simulink model "DAC_SIM_HL"  (R2017b)
settings: Solver=VariableStepDiscrete  StartTime=0.0  StopTime=N/Fs  RelTol=1e-3  EnableMultiTasking=on
values from neighbouring files (symbols this model uses):
  A = 0.5*(2-1)    (= 0.5)    [Model.m]
  ftest = 9e6    (= 9000000)    [Model.m]
  Tpass = 1/Fpass    (= 3.25520833333e-08)    [Model.m]
undefined symbols (not defined in the file or in its folder): a1, a2, a3, a4, b1, b2, b3, b4, g1, g2, g3, g4
libraries: dspmlti4 x3, dspsigops x2, simulink x1, dspsrcs4 x1
settings Model: Creator=o_cotte  LastModifiedBy=o_cotte
settings DataIOCC: LimitDataPoints=on  SaveFormat=Array
settings OptimizationCC: LifeSpan=inf
settings DebuggingCC: UnderspecifiedInitializationDetection=Classic  MergeDetectMultiDrivingBlocksExec=none  SolverPrmCheckMsg=warning  SFUnexpectedBacktrackingDiag=warning  SFNoUnconditionalDefaultTransitionDiag=warning  SFExecutionAtInitializationDiag=none
settings HardwareCC: ProdBitPerPointer=32  ProdBitPerSizeT=32  ProdBitPerPtrDiffT=32  ProdLargestAtomicFloat=None  ProdIntDivRoundTo=Undefined  ProdEndianess=Unspecified  ProdWordSize=32  ProdHWDeviceType=32-bit Generic
settings ModelReferenceCC: PropagateSignalLabelsOutOfModel=off
settings CodeAppCC: StateflowObjectComments=on
settings GRTTargetCC: TargetLangStandard=C89/C90 (ANSI)  GeneratePreprocessorConditionals=Disable all
settings ConfigComp: CovMetricSettings=dw  CovHtmlReporting=on  CovSaveCumulativeToWorkspaceVar=on  CovSaveSingleToWorkspaceVar=on  CovExternalEMLEnable=off

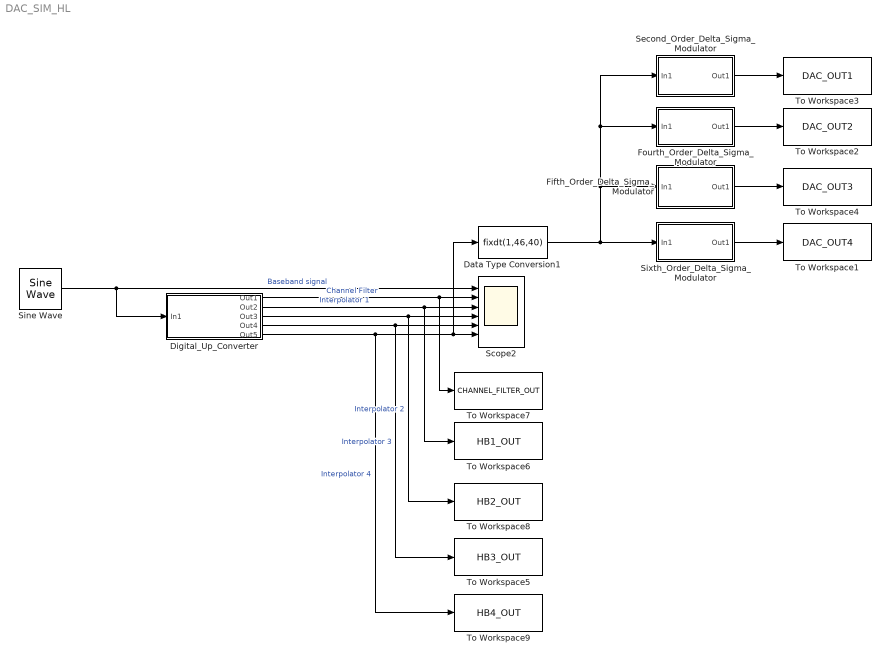
== system DAC_SIM_HL ==
  Data Type Conversion1 : DataTypeConversion  OutDataTypeStr=fixdt(1,46,40)  LockScale=on
  Digital_Up_Converter : Subsystem
  Fifth_Order_Delta_Sigma_Modulator : Subsystem
  Fourth_Order_Delta_Sigma_Modulator : Subsystem
  Scope2 : Scope  NumInputPorts=6
  Second_Order_Delta_Sigma_Modulator : Subsystem
  Sine Wave : dspsrcs4/Sine Wave  Amplitude=A  Frequency=ftest  Phase=0  SampleMode=Discrete  OutComplex=Real  CompMethod=Trigonometric fcn  TableSize=Speed  SampleTime=Tpass  SamplesPerFrame=1  ResetState=Restart at time zero  OutputFrames=on  dataType=double  wordLen=16  udDataType=sfix(16)  fracBitsMode=Best precision  numFracBits=15  OutDataTypeStr=double  LastOutDataTypeStr=double
  Sixth_Order_Delta_Sigma_Modulator : Subsystem
  To Workspace1 : ToWorkspace  VariableName=DAC_OUT4  SampleTime=-1
  To Workspace2 : ToWorkspace  VariableName=DAC_OUT2  SampleTime=-1
  To Workspace3 : ToWorkspace  VariableName=DAC_OUT1  SampleTime=-1
  To Workspace4 : ToWorkspace  VariableName=DAC_OUT3  SampleTime=-1
  To Workspace5 : ToWorkspace  VariableName=HB3_OUT  SampleTime=-1
  To Workspace6 : ToWorkspace  VariableName=HB1_OUT  SampleTime=-1
  To Workspace7 : ToWorkspace  VariableName=CHANNEL_FILTER_OUT  SampleTime=-1
  To Workspace8 : ToWorkspace  VariableName=HB2_OUT  SampleTime=-1
  To Workspace9 : ToWorkspace  VariableName=HB4_OUT  SampleTime=-1
  wires:
  Sine Wave/1 -> Digital_Up_Converter/1(In1), Scope2/1  "Baseband signal"
  Second_Order_Delta_Sigma_Modulator/1(Out1) -> To Workspace3/1
  Fourth_Order_Delta_Sigma_Modulator/1(Out1) -> To Workspace2/1
  Fifth_Order_Delta_Sigma_Modulator/1(Out1) -> To Workspace4/1
  Sixth_Order_Delta_Sigma_Modulator/1(Out1) -> To Workspace1/1
  Data Type Conversion1/1 -> Second_Order_Delta_Sigma_Modulator/1(In1), Fourth_Order_Delta_Sigma_Modulator/1(In1), Fifth_Order_Delta_Sigma_Modulator/1(In1), Sixth_Order_Delta_Sigma_Modulator/1(In1)
  Digital_Up_Converter/5(Out5) -> To Workspace9/1, Scope2/6, Data Type Conversion1/1  "Interpolator 4"
  Digital_Up_Converter/1(Out1) -> To Workspace7/1, Scope2/2  "Channel Filter"
  Digital_Up_Converter/2(Out2) -> To Workspace6/1, Scope2/3  "Interpolator 1"
  Digital_Up_Converter/3(Out3) -> To Workspace8/1, Scope2/4  "Interpolator 2"
  Digital_Up_Converter/4(Out4) -> To Workspace5/1, Scope2/5  "Interpolator 3"

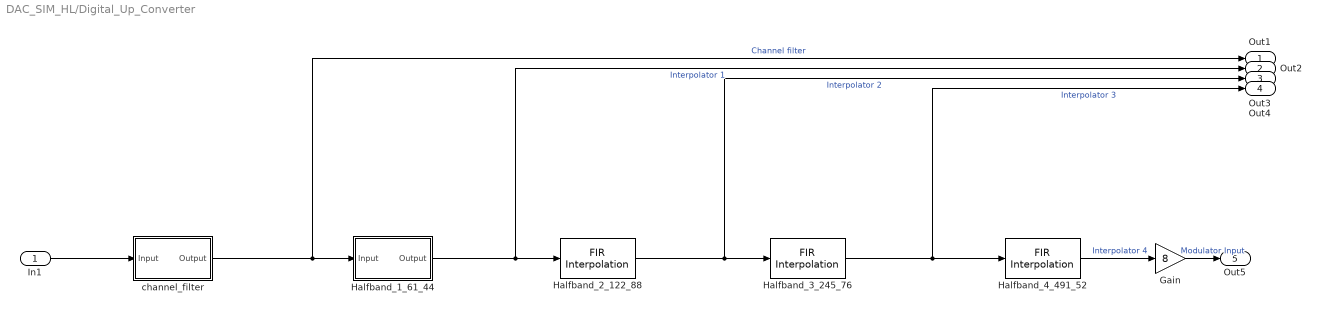
== system DAC_SIM_HL/Digital_Up_Converter ==
  In1 : Inport
  Gain : Gain  Gain=8
  Halfband_1_61_44 : Subsystem  Tag=FilterWizardSubSystem
      settings: ErrorFcn=dspFilterRealizedInBasicElemsAlgLoopErrFcnCallback
  Halfband_2_122_88 : dspmlti4/FIR Interpolation  Tag=BlockMethodSubSystem  FilterSource=Dialog parameters  h=[0.0076603622763803236 0 -0.053660411625164647 0 0.29602584582284724 0.5 0.29602584582284724 0 -0.053660411625164647 0 0.0076603622763803236]  L=2  FilterObject=Hm_firinterp  framing=Allow multirate processing  outputBufInitCond=0  roundingMode=Floor  overflowMode=off  firstCoeffDataTypeStr=Inherit: Same word length as input  firstCoeffMin=[]  firstCoeffMax=[]  firstCoeffLastDataTypeStr=Inherit: Same word length as input  outputDataTypeStr=Inherit: Same as accumulator  outputMin=[]  outputMax=[]  outputLastDataTypeStr=Inherit: Same as accumulator
      settings: SourceProductName=DSP System Toolbox
  Halfband_3_245_76 : dspmlti4/FIR Interpolation  Tag=BlockMethodSubSystem  FilterSource=Dialog parameters  h=[-0.032520171835777864 0 0.28248678153183715 0.5 0.28248678153183715 0 -0.032520171835777864]  L=2  FilterObject=Hm_firinterp  framing=Allow multirate processing  outputBufInitCond=0  roundingMode=Floor  overflowMode=off  firstCoeffDataTypeStr=Inherit: Same word length as input  firstCoeffMin=[]  firstCoeffMax=[]  firstCoeffLastDataTypeStr=Inherit: Same word length as input  outputDataTypeStr=Inherit: Same as accumulator  outputMin=[]  outputMax=[]  outputLastDataTypeStr=Inherit: Same as accumulator
      settings: SourceProductName=DSP System Toolbox
  Halfband_4_491_52 : dspmlti4/FIR Interpolation  Tag=BlockMethodSubSystem  FilterSource=Dialog parameters  h=[-0.031562027713033632 0 0.2815599679676668 0.5 0.2815599679676668 0 -0.031562027713033632]  L=2  FilterObject=Hm_firinterp  framing=Allow multirate processing  outputBufInitCond=0  roundingMode=Floor  overflowMode=off  firstCoeffDataTypeStr=Inherit: Same word length as input  firstCoeffMin=[]  firstCoeffMax=[]  firstCoeffLastDataTypeStr=Inherit: Same word length as input  outputDataTypeStr=Inherit: Same as accumulator  outputMin=[]  outputMax=[]  outputLastDataTypeStr=Inherit: Same as accumulator
      settings: SourceProductName=DSP System Toolbox
  channel_filter : Subsystem  Tag=FilterWizardSubSystem
      settings: ErrorFcn=dspFilterRealizedInBasicElemsAlgLoopErrFcnCallback
  Out1 : Outport
  Out2 : Outport  Port=2
  Out3 : Outport  Port=3
  Out4 : Outport  Port=4
  Out5 : Outport  Port=5
  wires:
  In1/1 -> channel_filter/1(Input)
  Halfband_1_61_44/1(Output) -> Out2/1, Halfband_2_122_88/1  "Interpolator 1"
  Halfband_2_122_88/1 -> Out3/1, Halfband_3_245_76/1  "Interpolator 2"
  Halfband_4_491_52/1 -> Gain/1  "Interpolator 4"
  Halfband_3_245_76/1 -> Out4/1, Halfband_4_491_52/1  "Interpolator 3"
  Gain/1 -> Out5/1  "Modulator Input"
  channel_filter/1(Output) -> Out1/1, Halfband_1_61_44/1(Input)  "Channel filter"

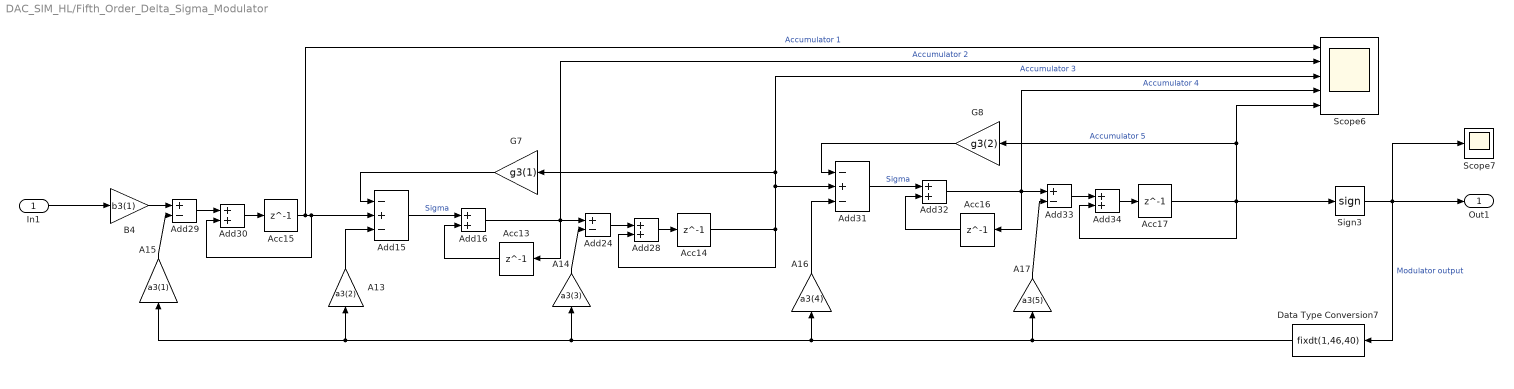
== system DAC_SIM_HL/Fifth_Order_Delta_Sigma_Modulator ==
  In1 : Inport
  A13 : Gain  Gain=a3(2)  OutDataTypeStr=Inherit: Same as input  ParamDataTypeStr=Inherit: Same as input  LockScale=on
  A14 : Gain  Gain=a3(3)  OutDataTypeStr=Inherit: Same as input  ParamDataTypeStr=Inherit: Same as input  LockScale=on
  A15 : Gain  Gain=a3(1)  OutDataTypeStr=Inherit: Same as input  ParamDataTypeStr=Inherit: Same as input  LockScale=on
  A16 : Gain  Gain=a3(4)  OutDataTypeStr=Inherit: Same as input  ParamDataTypeStr=Inherit: Same as input  LockScale=on
  A17 : Gain  Gain=a3(5)  OutDataTypeStr=Inherit: Same as input  ParamDataTypeStr=Inherit: Same as input  LockScale=on
  Acc{13..17} (5 alike) : Delay  DelayLength=1  InitialCondition=0
  Add15 : Sum  Inputs=-+-  SaturateOnIntegerOverflow=on  InputSameDT=on  OutDataTypeStr=Inherit: Same as first input
  Add{16,28,30,32,34} (5 alike) : Sum  Inputs=2  SaturateOnIntegerOverflow=on  InputSameDT=on  OutDataTypeStr=Inherit: Same as first input
  Add24 : Sum  Inputs=+-  SaturateOnIntegerOverflow=on  InputSameDT=on  OutDataTypeStr=Inherit: Same as first input
  Add29 : Sum  Inputs=+-  SaturateOnIntegerOverflow=on  InputSameDT=on  OutDataTypeStr=Inherit: Same as first input
  Add31 : Sum  Inputs=-+-  SaturateOnIntegerOverflow=on  InputSameDT=on  OutDataTypeStr=Inherit: Same as first input
  Add33 : Sum  Inputs=+-  SaturateOnIntegerOverflow=on  InputSameDT=on  OutDataTypeStr=Inherit: Same as first input
  B4 : Gain  Gain=b3(1)  OutDataTypeStr=Inherit: Same as input  ParamDataTypeStr=Inherit: Same as input  LockScale=on
  Data Type Conversion7 : DataTypeConversion  OutDataTypeStr=fixdt(1,46,40)  LockScale=on
  G7 : Gain  Gain=g3(1)  OutDataTypeStr=Inherit: Same as input  ParamDataTypeStr=Inherit: Same as input  LockScale=on
  G8 : Gain  Gain=g3(2)  OutDataTypeStr=Inherit: Same as input  ParamDataTypeStr=Inherit: Same as input  LockScale=on
  Scope6 : Scope  NumInputPorts=5
  Scope7 : Scope
  Sign3 : Signum
  Out1 : Outport
  wires:
  Acc16/1 -> Add32/2
  A16/1 -> Add31/3
  Add33/1 -> Add34/1
  G8/1 -> Add31/1
  Data Type Conversion7/1 -> A17/1, A14/1, A15/1, A13/1, A16/1
  A17/1 -> Add33/2
  Add31/1 -> Add32/1  "Sigma"
  Acc17/1 -> Sign3/1, Add34/2, Scope6/5, G8/1  "Accumulator 5"
  Add32/1 -> Scope6/4, Add33/1, Acc16/1  "Accumulator 4"
  Add34/1 -> Acc17/1
  Add24/1 -> Add28/1
  Acc13/1 -> Add16/2
  Add29/1 -> Add30/1
  Add30/1 -> Acc15/1
  A13/1 -> Add15/3
  Sign3/1 -> Scope7/1, Out1/1, Data Type Conversion7/1  "Modulator output"
  In1/1 -> B4/1
  Add16/1 -> Scope6/2, Add24/1, Acc13/1  "Accumulator 2"
  A15/1 -> Add29/2
  G7/1 -> Add15/1
  Acc14/1 -> Add31/2, Scope6/3, G7/1, Add28/2  "Accumulator 3"
  Add28/1 -> Acc14/1
  A14/1 -> Add24/2
  Acc15/1 -> Scope6/1, Add15/2, Add30/2  "Accumulator 1"
  Add15/1 -> Add16/1  "Sigma"
  B4/1 -> Add29/1

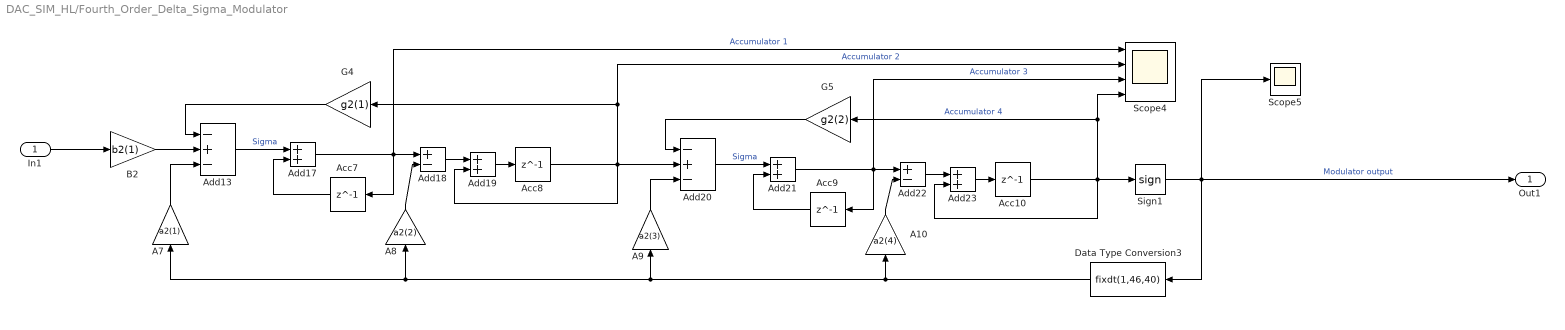
== system DAC_SIM_HL/Fourth_Order_Delta_Sigma_Modulator ==
  In1 : Inport
  A10 : Gain  Gain=a2(4)  OutDataTypeStr=Inherit: Same as input  ParamDataTypeStr=Inherit: Same as input  LockScale=on
  A7 : Gain  Gain=a2(1)  OutDataTypeStr=Inherit: Same as input  ParamDataTypeStr=Inherit: Same as input  LockScale=on
  A8 : Gain  Gain=a2(2)  OutDataTypeStr=Inherit: Same as input  ParamDataTypeStr=Inherit: Same as input  LockScale=on
  A9 : Gain  Gain=a2(3)  OutDataTypeStr=Inherit: Same as input  ParamDataTypeStr=Inherit: Same as input  LockScale=on
  Acc{7..10} (4 alike) : Delay  DelayLength=1  InitialCondition=0
  Add13 : Sum  Inputs=-+-  SaturateOnIntegerOverflow=on  InputSameDT=on  OutDataTypeStr=Inherit: Same as first input
  Add{17,19,21,23} (4 alike) : Sum  Inputs=2  SaturateOnIntegerOverflow=on  InputSameDT=on  OutDataTypeStr=Inherit: Same as first input
  Add18 : Sum  Inputs=+-  SaturateOnIntegerOverflow=on  InputSameDT=on  OutDataTypeStr=Inherit: Same as first input
  Add20 : Sum  Inputs=-+-  SaturateOnIntegerOverflow=on  InputSameDT=on  OutDataTypeStr=Inherit: Same as first input
  Add22 : Sum  Inputs=+-  SaturateOnIntegerOverflow=on  InputSameDT=on  OutDataTypeStr=Inherit: Same as first input
  B2 : Gain  Gain=b2(1)  OutDataTypeStr=Inherit: Same as input  ParamDataTypeStr=Inherit: Same as input  LockScale=on
  Data Type Conversion3 : DataTypeConversion  OutDataTypeStr=fixdt(1,46,40)  LockScale=on
  G4 : Gain  Gain=g2(1)  OutDataTypeStr=Inherit: Same as input  ParamDataTypeStr=Inherit: Same as input  LockScale=on
  G5 : Gain  Gain=g2(2)  OutDataTypeStr=Inherit: Same as input  ParamDataTypeStr=Inherit: Same as input  LockScale=on
  Scope4 : Scope  NumInputPorts=4
  Scope5 : Scope
  Sign1 : Signum
  Out1 : Outport
  wires:
  Sign1/1 -> Out1/1, Data Type Conversion3/1, Scope5/1  "Modulator output"
  Add13/1 -> Add17/1  "Sigma"
  In1/1 -> B2/1
  Data Type Conversion3/1 -> A10/1, A9/1, A7/1, A8/1
  B2/1 -> Add13/2
  Add17/1 -> Scope4/1, Add18/1, Acc7/1  "Accumulator 1"
  Acc8/1 -> Add20/2, Add19/2, Scope4/2, G4/1  "Accumulator 2"
  A7/1 -> Add13/3
  Acc7/1 -> Add17/2
  Acc10/1 -> Sign1/1, Scope4/4, G5/1, Add23/2  "Accumulator 4"
  Add19/1 -> Acc8/1
  Add18/1 -> Add19/1
  Add22/1 -> Add23/1
  G5/1 -> Add20/1
  Add23/1 -> Acc10/1
  Add21/1 -> Acc9/1, Scope4/3, Add22/1  "Accumulator 3"
  A10/1 -> Add22/2
  A8/1 -> Add18/2
  A9/1 -> Add20/3
  G4/1 -> Add13/1
  Add20/1 -> Add21/1  "Sigma"
  Acc9/1 -> Add21/2

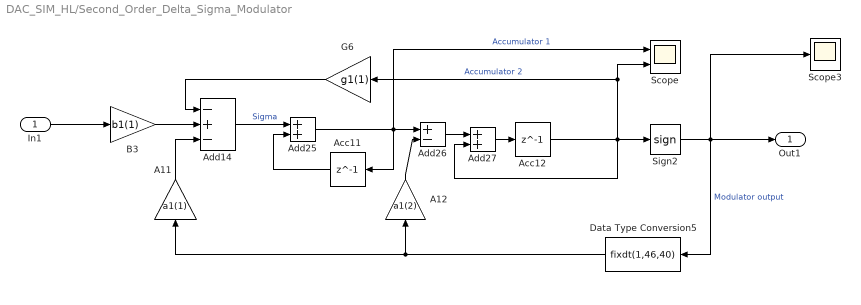
== system DAC_SIM_HL/Second_Order_Delta_Sigma_Modulator ==
  In1 : Inport
  A11 : Gain  Gain=a1(1)  OutDataTypeStr=Inherit: Same as input  ParamDataTypeStr=Inherit: Same as input  LockScale=on
  A12 : Gain  Gain=a1(2)  OutDataTypeStr=Inherit: Same as input  ParamDataTypeStr=Inherit: Same as input  LockScale=on
  Acc11 : Delay  DelayLength=1  InitialCondition=0
  Acc12 : Delay  DelayLength=1  InitialCondition=0
  Add14 : Sum  Inputs=-+-  SaturateOnIntegerOverflow=on  InputSameDT=on  OutDataTypeStr=Inherit: Same as first input
  Add25 : Sum  Inputs=2  SaturateOnIntegerOverflow=on  InputSameDT=on  OutDataTypeStr=Inherit: Same as first input
  Add26 : Sum  Inputs=+-  SaturateOnIntegerOverflow=on  InputSameDT=on  OutDataTypeStr=Inherit: Same as first input
  Add27 : Sum  Inputs=2  SaturateOnIntegerOverflow=on  InputSameDT=on  OutDataTypeStr=Inherit: Same as first input
  B3 : Gain  Gain=b1(1)  OutDataTypeStr=Inherit: Same as input  ParamDataTypeStr=Inherit: Same as input  LockScale=on
  Data Type Conversion5 : DataTypeConversion  OutDataTypeStr=fixdt(1,46,40)  LockScale=on
  G6 : Gain  Gain=g1(1)  OutDataTypeStr=Inherit: Same as input  ParamDataTypeStr=Inherit: Same as input  LockScale=on
  Scope : Scope  NumInputPorts=2
  Scope3 : Scope
  Sign2 : Signum
  Out1 : Outport
  wires:
  Data Type Conversion5/1 -> A12/1, A11/1
  A11/1 -> Add14/3
  G6/1 -> Add14/1
  B3/1 -> Add14/2
  Acc11/1 -> Add25/2
  Add25/1 -> Scope/1, Add26/1, Acc11/1  "Accumulator 1"
  Acc12/1 -> Sign2/1, Add27/2, Scope/2, G6/1  "Accumulator 2"
  Add27/1 -> Acc12/1
  A12/1 -> Add26/2
  Add26/1 -> Add27/1
  In1/1 -> B3/1
  Add14/1 -> Add25/1  "Sigma"
  Sign2/1 -> Out1/1, Scope3/1, Data Type Conversion5/1  "Modulator output"

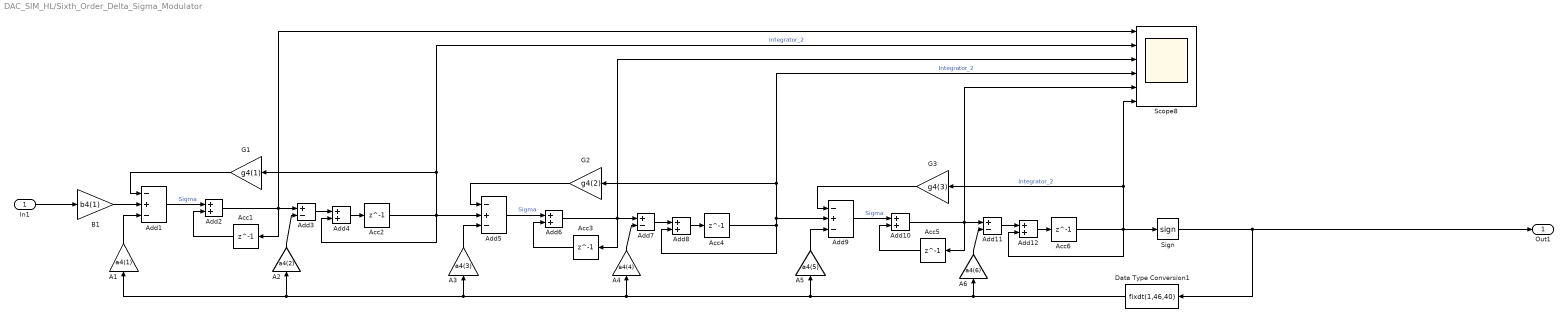
== system DAC_SIM_HL/Sixth_Order_Delta_Sigma_Modulator ==
  In1 : Inport
  A1 : Gain  Gain=a4(1)  OutDataTypeStr=Inherit: Same as input  ParamDataTypeStr=Inherit: Same as input  LockScale=on
  A2 : Gain  Gain=a4(2)  OutDataTypeStr=Inherit: Same as input  ParamDataTypeStr=Inherit: Same as input  LockScale=on
  A3 : Gain  Gain=a4(3)  OutDataTypeStr=Inherit: Same as input  ParamDataTypeStr=Inherit: Same as input  LockScale=on
  A4 : Gain  Gain=a4(4)  OutDataTypeStr=Inherit: Same as input  ParamDataTypeStr=Inherit: Same as input  LockScale=on
  A5 : Gain  Gain=a4(5)  OutDataTypeStr=Inherit: Same as input  ParamDataTypeStr=Inherit: Same as input  LockScale=on
  A6 : Gain  Gain=a4(6)  OutDataTypeStr=Inherit: Same as input  ParamDataTypeStr=Inherit: Same as input  LockScale=on
  Acc{1..6} (6 alike) : Delay  DelayLength=1  InitialCondition=0
  Add1 : Sum  Inputs=-+-  SaturateOnIntegerOverflow=on  InputSameDT=on  OutDataTypeStr=Inherit: Same as first input
  Add{2,4,6,8,10,12} (6 alike) : Sum  Inputs=2  SaturateOnIntegerOverflow=on  InputSameDT=on  OutDataTypeStr=Inherit: Same as first input
  Add11 : Sum  Inputs=+-  SaturateOnIntegerOverflow=on  InputSameDT=on  OutDataTypeStr=Inherit: Same as first input
  Add3 : Sum  Inputs=+-  SaturateOnIntegerOverflow=on  InputSameDT=on  OutDataTypeStr=Inherit: Same as first input
  Add5 : Sum  Inputs=-+-  SaturateOnIntegerOverflow=on  InputSameDT=on  OutDataTypeStr=Inherit: Same as first input
  Add7 : Sum  Inputs=+-  SaturateOnIntegerOverflow=on  InputSameDT=on  OutDataTypeStr=Inherit: Same as first input
  Add9 : Sum  Inputs=-+-  SaturateOnIntegerOverflow=on  InputSameDT=on  OutDataTypeStr=Inherit: Same as first input
  B1 : Gain  Gain=b4(1)  OutDataTypeStr=Inherit: Same as input  ParamDataTypeStr=Inherit: Same as input  LockScale=on
  Data Type Conversion1 : DataTypeConversion  OutDataTypeStr=fixdt(1,46,40)  LockScale=on
  G1 : Gain  Gain=g4(1)  OutDataTypeStr=Inherit: Same as input  ParamDataTypeStr=Inherit: Same as input  LockScale=on
  G2 : Gain  Gain=g4(2)  OutDataTypeStr=Inherit: Same as input  ParamDataTypeStr=Inherit: Same as input  LockScale=on
  G3 : Gain  Gain=g4(3)  OutDataTypeStr=Inherit: Same as input  ParamDataTypeStr=Inherit: Same as input  LockScale=on
  Scope8 : Scope  NumInputPorts=6
  Sign : Signum
  Out1 : Outport
  wires:
  Add1/1 -> Add2/1  "Sigma"
  Sign/1 -> Out1/1, Data Type Conversion1/1
  In1/1 -> B1/1
  Data Type Conversion1/1 -> A6/1, A4/1, A1/1, A2/1, A3/1, A5/1
  B1/1 -> Add1/2
  A1/1 -> Add1/3
  Acc1/1 -> Add2/2
  Add2/1 -> Scope8/1, Add3/1, Acc1/1
  Add4/1 -> Acc2/1
  G1/1 -> Add1/1
  Acc2/1 -> Add5/2, Add4/2, Scope8/2, G1/1  "Integrator_2"
  Add3/1 -> Add4/1
  A2/1 -> Add3/2
  Add5/1 -> Add6/1  "Sigma"
  A3/1 -> Add5/3
  Add11/1 -> Add12/1
  G3/1 -> Add9/1
  Add6/1 -> Scope8/3, Add7/1, Acc3/1
  A6/1 -> Add11/2
  Acc3/1 -> Add6/2
  Acc4/1 -> Add9/2, Scope8/4, G2/1, Add8/2  "Integrator_2"
  Add9/1 -> Add10/1  "Sigma"
  Add7/1 -> Add8/1
  A5/1 -> Add9/3
  Add10/1 -> Scope8/5, Add11/1, Acc5/1
  Add12/1 -> Acc6/1
  Acc6/1 -> Sign/1, Add12/2, Scope8/6, G3/1  "Integrator_2"
  Acc5/1 -> Add10/2
  Add8/1 -> Acc4/1
  G2/1 -> Add5/1
  A4/1 -> Add7/2

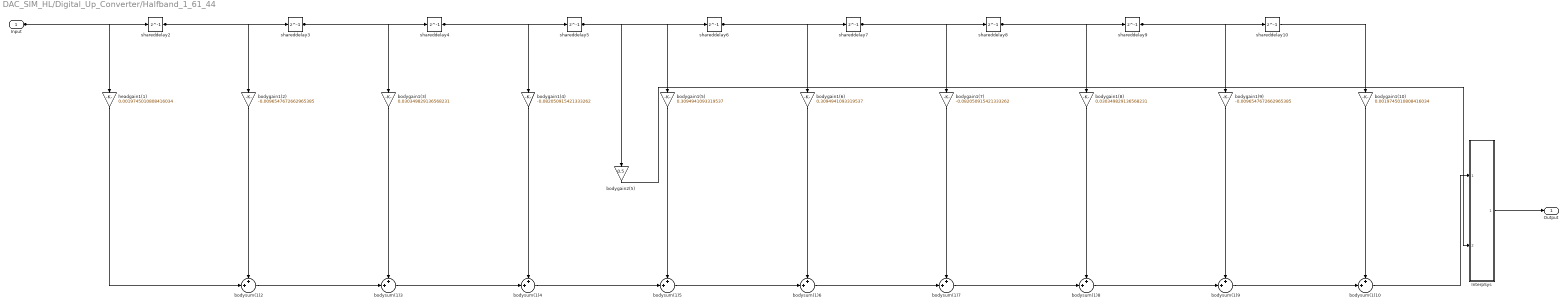
== system DAC_SIM_HL/Digital_Up_Converter/Halfband_1_61_44 ==
  Input : Inport
  InterpSys : Subsystem  Tag=FilterWizardInterpolatorCommutator
  bodygain1(10) : Gain  Gain=0.0019745010808416034  ParamDataTypeStr=double  RndMeth=Nearest  SaturateOnIntegerOverflow=on  OutDataTypeStr=Inherit: Same as input
  bodygain1(2) : Gain  Gain=-0.0096547672662965385  ParamDataTypeStr=double  RndMeth=Nearest  SaturateOnIntegerOverflow=on  OutDataTypeStr=Inherit: Same as input
  bodygain1(3) : Gain  Gain=0.030349829136568231  ParamDataTypeStr=double  RndMeth=Nearest  SaturateOnIntegerOverflow=on  OutDataTypeStr=Inherit: Same as input
  bodygain1(4) : Gain  Gain=-0.082050915421333262  ParamDataTypeStr=double  RndMeth=Nearest  SaturateOnIntegerOverflow=on  OutDataTypeStr=Inherit: Same as input
  bodygain1(5) : Gain  Gain=0.3094941093319537  ParamDataTypeStr=double  RndMeth=Nearest  SaturateOnIntegerOverflow=on  OutDataTypeStr=Inherit: Same as input
  bodygain1(6) : Gain  Gain=0.3094941093319537  ParamDataTypeStr=double  RndMeth=Nearest  SaturateOnIntegerOverflow=on  OutDataTypeStr=Inherit: Same as input
  bodygain1(7) : Gain  Gain=-0.082050915421333262  ParamDataTypeStr=double  RndMeth=Nearest  SaturateOnIntegerOverflow=on  OutDataTypeStr=Inherit: Same as input
  bodygain1(8) : Gain  Gain=0.030349829136568231  ParamDataTypeStr=double  RndMeth=Nearest  SaturateOnIntegerOverflow=on  OutDataTypeStr=Inherit: Same as input
  bodygain1(9) : Gain  Gain=-0.0096547672662965385  ParamDataTypeStr=double  RndMeth=Nearest  SaturateOnIntegerOverflow=on  OutDataTypeStr=Inherit: Same as input
  bodygain2(5) : Gain  Gain=0.5  ParamDataTypeStr=double  RndMeth=Nearest  SaturateOnIntegerOverflow=on  OutDataTypeStr=Inherit: Same as input
  bodysum(1){2..10} (9 alike) : Sum  Inputs=++|  RndMeth=Nearest  SaturateOnIntegerOverflow=on  OutDataTypeStr=Inherit: Same as first input
  headgain1(1) : Gain  Gain=0.0019745010808416034  ParamDataTypeStr=double  RndMeth=Nearest  SaturateOnIntegerOverflow=on  OutDataTypeStr=Inherit: Same as input
  shareddelay{2..10} (9 alike) : Delay  DelayLength=1  InitialCondition=0
  Output : Outport
  wires:
  headgain1(1)/1 -> bodysum(1)2/2
  Input/1 -> headgain1(1)/1, shareddelay2/1
  bodygain1(2)/1 -> bodysum(1)2/1
  bodysum(1)2/1 -> bodysum(1)3/2
  shareddelay2/1 -> bodygain1(2)/1, shareddelay3/1
  bodygain1(3)/1 -> bodysum(1)3/1
  bodysum(1)3/1 -> bodysum(1)4/2
  shareddelay3/1 -> bodygain1(3)/1, shareddelay4/1
  bodygain1(4)/1 -> bodysum(1)4/1
  bodysum(1)4/1 -> bodysum(1)5/2
  shareddelay4/1 -> bodygain1(4)/1, shareddelay5/1
  bodygain1(5)/1 -> bodysum(1)5/1
  bodygain2(5)/1 -> InterpSys/2(input2)
  bodysum(1)5/1 -> bodysum(1)6/2
  shareddelay5/1 -> bodygain1(5)/1, bodygain2(5)/1, shareddelay6/1
  bodygain1(6)/1 -> bodysum(1)6/1
  bodysum(1)6/1 -> bodysum(1)7/2
  shareddelay6/1 -> bodygain1(6)/1, shareddelay7/1
  bodygain1(7)/1 -> bodysum(1)7/1
  bodysum(1)7/1 -> bodysum(1)8/2
  shareddelay7/1 -> bodygain1(7)/1, shareddelay8/1
  bodygain1(8)/1 -> bodysum(1)8/1
  bodysum(1)8/1 -> bodysum(1)9/2
  shareddelay8/1 -> bodygain1(8)/1, shareddelay9/1
  bodygain1(9)/1 -> bodysum(1)9/1
  bodysum(1)9/1 -> bodysum(1)10/2
  shareddelay9/1 -> bodygain1(9)/1, shareddelay10/1
  bodygain1(10)/1 -> bodysum(1)10/1
  bodysum(1)10/1 -> InterpSys/1(input1)
  shareddelay10/1 -> bodygain1(10)/1
  InterpSys/1(output) -> Output/1

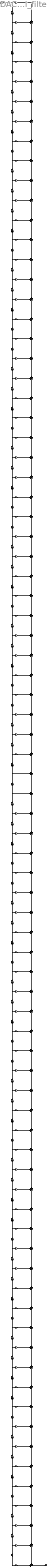
== system DAC_SIM_HL/Digital_Up_Converter/channel_filter ==
  Input : Inport
  BodyDelay{2..80} (79 alike) : Delay  DelayLength=1  InitialCondition=0
  BodyLSum{2..80} (79 alike) : Sum  Inputs=++|  RndMeth=Nearest  SaturateOnIntegerOverflow=on  OutDataTypeStr=Inherit: Same as first input
  b(1) : Gain  Gain=0.001967203062125656  ParamDataTypeStr=double  RndMeth=Nearest  SaturateOnIntegerOverflow=on  OutDataTypeStr=Inherit: Same as input
  b(10) : Gain  Gain=0.0012499054459363052  ParamDataTypeStr=double  RndMeth=Nearest  SaturateOnIntegerOverflow=on  OutDataTypeStr=Inherit: Same as input
  b(11) : Gain  Gain=0.0063779584212783945  ParamDataTypeStr=double  RndMeth=Nearest  SaturateOnIntegerOverflow=on  OutDataTypeStr=Inherit: Same as input
  b(12) : Gain  Gain=-0.006863487310719423  ParamDataTypeStr=double  RndMeth=Nearest  SaturateOnIntegerOverflow=on  OutDataTypeStr=Inherit: Same as input
  b(13) : Gain  Gain=-0.0022149724080229262  ParamDataTypeStr=double  RndMeth=Nearest  SaturateOnIntegerOverflow=on  OutDataTypeStr=Inherit: Same as input
  b(14) : Gain  Gain=0.010309848768947499  ParamDataTypeStr=double  RndMeth=Nearest  SaturateOnIntegerOverflow=on  OutDataTypeStr=Inherit: Same as input
  b(15) : Gain  Gain=-0.0057995752256193292  ParamDataTypeStr=double  RndMeth=Nearest  SaturateOnIntegerOverflow=on  OutDataTypeStr=Inherit: Same as input
  b(16) : Gain  Gain=-0.0078393747460676639  ParamDataTypeStr=double  RndMeth=Nearest  SaturateOnIntegerOverflow=on  OutDataTypeStr=Inherit: Same as input
  b(17) : Gain  Gain=0.013515839977527713  ParamDataTypeStr=double  RndMeth=Nearest  SaturateOnIntegerOverflow=on  OutDataTypeStr=Inherit: Same as input
  b(18) : Gain  Gain=-0.0015560228112558043  ParamDataTypeStr=double  RndMeth=Nearest  SaturateOnIntegerOverflow=on  OutDataTypeStr=Inherit: Same as input
  b(19) : Gain  Gain=-0.0151258138642529  ParamDataTypeStr=double  RndMeth=Nearest  SaturateOnIntegerOverflow=on  OutDataTypeStr=Inherit: Same as input
  b(2) : Gain  Gain=0.0014942521610644595  ParamDataTypeStr=double  RndMeth=Nearest  SaturateOnIntegerOverflow=on  OutDataTypeStr=Inherit: Same as input
  b(20) : Gain  Gain=0.014256849182145013  ParamDataTypeStr=double  RndMeth=Nearest  SaturateOnIntegerOverflow=on  OutDataTypeStr=Inherit: Same as input
  b(21) : Gain  Gain=0.0066509239213464093  ParamDataTypeStr=double  RndMeth=Nearest  SaturateOnIntegerOverflow=on  OutDataTypeStr=Inherit: Same as input
  b(22) : Gain  Gain=-0.022673125747107812  ParamDataTypeStr=double  RndMeth=Nearest  SaturateOnIntegerOverflow=on  OutDataTypeStr=Inherit: Same as input
  b(23) : Gain  Gain=0.010467912906156281  ParamDataTypeStr=double  RndMeth=Nearest  SaturateOnIntegerOverflow=on  OutDataTypeStr=Inherit: Same as input
  b(24) : Gain  Gain=0.018904809782294026  ParamDataTypeStr=double  RndMeth=Nearest  SaturateOnIntegerOverflow=on  OutDataTypeStr=Inherit: Same as input
  b(25) : Gain  Gain=-0.028151945611142579  ParamDataTypeStr=double  RndMeth=Nearest  SaturateOnIntegerOverflow=on  OutDataTypeStr=Inherit: Same as input
  b(26) : Gain  Gain=3.7719500840953233e-05  ParamDataTypeStr=double  RndMeth=Nearest  SaturateOnIntegerOverflow=on  OutDataTypeStr=Inherit: Same as input
  b(27) : Gain  Gain=0.034369057437976067  ParamDataTypeStr=double  RndMeth=Nearest  SaturateOnIntegerOverflow=on  OutDataTypeStr=Inherit: Same as input
  b(28) : Gain  Gain=-0.028320189372389365  ParamDataTypeStr=double  RndMeth=Nearest  SaturateOnIntegerOverflow=on  OutDataTypeStr=Inherit: Same as input
  b(29) : Gain  Gain=-0.019152553334523169  ParamDataTypeStr=double  RndMeth=Nearest  SaturateOnIntegerOverflow=on  OutDataTypeStr=Inherit: Same as input
  b(3) : Gain  Gain=-0.0040029332081024669  ParamDataTypeStr=double  RndMeth=Nearest  SaturateOnIntegerOverflow=on  OutDataTypeStr=Inherit: Same as input
  b(30) : Gain  Gain=0.051285882661541167  ParamDataTypeStr=double  RndMeth=Nearest  SaturateOnIntegerOverflow=on  OutDataTypeStr=Inherit: Same as input
  b(31) : Gain  Gain=-0.018627713050824883  ParamDataTypeStr=double  RndMeth=Nearest  SaturateOnIntegerOverflow=on  OutDataTypeStr=Inherit: Same as input
  b(32) : Gain  Gain=-0.050211030664596111  ParamDataTypeStr=double  RndMeth=Nearest  SaturateOnIntegerOverflow=on  OutDataTypeStr=Inherit: Same as input
  b(33) : Gain  Gain=0.067266164111800655  ParamDataTypeStr=double  RndMeth=Nearest  SaturateOnIntegerOverflow=on  OutDataTypeStr=Inherit: Same as input
  b(34) : Gain  Gain=0.0094569817819130635  ParamDataTypeStr=double  RndMeth=Nearest  SaturateOnIntegerOverflow=on  OutDataTypeStr=Inherit: Same as input
  b(35) : Gain  Gain=-0.10259153598421479  ParamDataTypeStr=double  RndMeth=Nearest  SaturateOnIntegerOverflow=on  OutDataTypeStr=Inherit: Same as input
  b(36) : Gain  Gain=0.079752718239406911  ParamDataTypeStr=double  RndMeth=Nearest  SaturateOnIntegerOverflow=on  OutDataTypeStr=Inherit: Same as input
  b(37) : Gain  Gain=0.087741449620747772  ParamDataTypeStr=double  RndMeth=Nearest  SaturateOnIntegerOverflow=on  OutDataTypeStr=Inherit: Same as input
  b(38) : Gain  Gain=-0.23705587106831169  ParamDataTypeStr=double  RndMeth=Nearest  SaturateOnIntegerOverflow=on  OutDataTypeStr=Inherit: Same as input
  b(39) : Gain  Gain=0.086606981592638604  ParamDataTypeStr=double  RndMeth=Nearest  SaturateOnIntegerOverflow=on  OutDataTypeStr=Inherit: Same as input
  b(4) : Gain  Gain=0.0039010037547926465  ParamDataTypeStr=double  RndMeth=Nearest  SaturateOnIntegerOverflow=on  OutDataTypeStr=Inherit: Same as input
  b(42) : Gain  Gain=0.086606981592638604  ParamDataTypeStr=double  RndMeth=Nearest  SaturateOnIntegerOverflow=on  OutDataTypeStr=Inherit: Same as input
  b(43) : Gain  Gain=-0.23705587106831169  ParamDataTypeStr=double  RndMeth=Nearest  SaturateOnIntegerOverflow=on  OutDataTypeStr=Inherit: Same as input
  b(44) : Gain  Gain=0.087741449620747772  ParamDataTypeStr=double  RndMeth=Nearest  SaturateOnIntegerOverflow=on  OutDataTypeStr=Inherit: Same as input
  b(45) : Gain  Gain=0.079752718239406911  ParamDataTypeStr=double  RndMeth=Nearest  SaturateOnIntegerOverflow=on  OutDataTypeStr=Inherit: Same as input
  b(46) : Gain  Gain=-0.10259153598421479  ParamDataTypeStr=double  RndMeth=Nearest  SaturateOnIntegerOverflow=on  OutDataTypeStr=Inherit: Same as input
  b(47) : Gain  Gain=0.0094569817819130635  ParamDataTypeStr=double  RndMeth=Nearest  SaturateOnIntegerOverflow=on  OutDataTypeStr=Inherit: Same as input
  b(48) : Gain  Gain=0.067266164111800655  ParamDataTypeStr=double  RndMeth=Nearest  SaturateOnIntegerOverflow=on  OutDataTypeStr=Inherit: Same as input
  b(49) : Gain  Gain=-0.050211030664596111  ParamDataTypeStr=double  RndMeth=Nearest  SaturateOnIntegerOverflow=on  OutDataTypeStr=Inherit: Same as input
  b(5) : Gain  Gain=-2.8914777875554402e-07  ParamDataTypeStr=double  RndMeth=Nearest  SaturateOnIntegerOverflow=on  OutDataTypeStr=Inherit: Same as input
  b(50) : Gain  Gain=-0.018627713050824883  ParamDataTypeStr=double  RndMeth=Nearest  SaturateOnIntegerOverflow=on  OutDataTypeStr=Inherit: Same as input
  b(51) : Gain  Gain=0.051285882661541167  ParamDataTypeStr=double  RndMeth=Nearest  SaturateOnIntegerOverflow=on  OutDataTypeStr=Inherit: Same as input
  b(52) : Gain  Gain=-0.019152553334523169  ParamDataTypeStr=double  RndMeth=Nearest  SaturateOnIntegerOverflow=on  OutDataTypeStr=Inherit: Same as input
  b(53) : Gain  Gain=-0.028320189372389365  ParamDataTypeStr=double  RndMeth=Nearest  SaturateOnIntegerOverflow=on  OutDataTypeStr=Inherit: Same as input
  b(54) : Gain  Gain=0.034369057437976067  ParamDataTypeStr=double  RndMeth=Nearest  SaturateOnIntegerOverflow=on  OutDataTypeStr=Inherit: Same as input
  b(55) : Gain  Gain=3.7719500840953233e-05  ParamDataTypeStr=double  RndMeth=Nearest  SaturateOnIntegerOverflow=on  OutDataTypeStr=Inherit: Same as input
  b(56) : Gain  Gain=-0.028151945611142579  ParamDataTypeStr=double  RndMeth=Nearest  SaturateOnIntegerOverflow=on  OutDataTypeStr=Inherit: Same as input
  b(57) : Gain  Gain=0.018904809782294026  ParamDataTypeStr=double  RndMeth=Nearest  SaturateOnIntegerOverflow=on  OutDataTypeStr=Inherit: Same as input
  b(58) : Gain  Gain=0.010467912906156281  ParamDataTypeStr=double  RndMeth=Nearest  SaturateOnIntegerOverflow=on  OutDataTypeStr=Inherit: Same as input
  b(59) : Gain  Gain=-0.022673125747107812  ParamDataTypeStr=double  RndMeth=Nearest  SaturateOnIntegerOverflow=on  OutDataTypeStr=Inherit: Same as input
  b(6) : Gain  Gain=-0.0038298703556784923  ParamDataTypeStr=double  RndMeth=Nearest  SaturateOnIntegerOverflow=on  OutDataTypeStr=Inherit: Same as input
  b(60) : Gain  Gain=0.0066509239213464093  ParamDataTypeStr=double  RndMeth=Nearest  SaturateOnIntegerOverflow=on  OutDataTypeStr=Inherit: Same as input
  b(61) : Gain  Gain=0.014256849182145013  ParamDataTypeStr=double  RndMeth=Nearest  SaturateOnIntegerOverflow=on  OutDataTypeStr=Inherit: Same as input
  b(62) : Gain  Gain=-0.0151258138642529  ParamDataTypeStr=double  RndMeth=Nearest  SaturateOnIntegerOverflow=on  OutDataTypeStr=Inherit: Same as input
  b(63) : Gain  Gain=-0.0015560228112558043  ParamDataTypeStr=double  RndMeth=Nearest  SaturateOnIntegerOverflow=on  OutDataTypeStr=Inherit: Same as input
  b(64) : Gain  Gain=0.013515839977527713  ParamDataTypeStr=double  RndMeth=Nearest  SaturateOnIntegerOverflow=on  OutDataTypeStr=Inherit: Same as input
  b(65) : Gain  Gain=-0.0078393747460676639  ParamDataTypeStr=double  RndMeth=Nearest  SaturateOnIntegerOverflow=on  OutDataTypeStr=Inherit: Same as input
  b(66) : Gain  Gain=-0.0057995752256193292  ParamDataTypeStr=double  RndMeth=Nearest  SaturateOnIntegerOverflow=on  OutDataTypeStr=Inherit: Same as input
  b(67) : Gain  Gain=0.010309848768947499  ParamDataTypeStr=double  RndMeth=Nearest  SaturateOnIntegerOverflow=on  OutDataTypeStr=Inherit: Same as input
  b(68) : Gain  Gain=-0.0022149724080229262  ParamDataTypeStr=double  RndMeth=Nearest  SaturateOnIntegerOverflow=on  OutDataTypeStr=Inherit: Same as input
  b(69) : Gain  Gain=-0.006863487310719423  ParamDataTypeStr=double  RndMeth=Nearest  SaturateOnIntegerOverflow=on  OutDataTypeStr=Inherit: Same as input
  b(7) : Gain  Gain=0.0025952474609302373  ParamDataTypeStr=double  RndMeth=Nearest  SaturateOnIntegerOverflow=on  OutDataTypeStr=Inherit: Same as input
  b(70) : Gain  Gain=0.0063779584212783945  ParamDataTypeStr=double  RndMeth=Nearest  SaturateOnIntegerOverflow=on  OutDataTypeStr=Inherit: Same as input
  b(71) : Gain  Gain=0.0012499054459363052  ParamDataTypeStr=double  RndMeth=Nearest  SaturateOnIntegerOverflow=on  OutDataTypeStr=Inherit: Same as input
  b(72) : Gain  Gain=-0.0059345211567351126  ParamDataTypeStr=double  RndMeth=Nearest  SaturateOnIntegerOverflow=on  OutDataTypeStr=Inherit: Same as input
  b(73) : Gain  Gain=0.002993986641238823  ParamDataTypeStr=double  RndMeth=Nearest  SaturateOnIntegerOverflow=on  OutDataTypeStr=Inherit: Same as input
  b(74) : Gain  Gain=0.0025952474609302373  ParamDataTypeStr=double  RndMeth=Nearest  SaturateOnIntegerOverflow=on  OutDataTypeStr=Inherit: Same as input
  b(75) : Gain  Gain=-0.0038298703556784923  ParamDataTypeStr=double  RndMeth=Nearest  SaturateOnIntegerOverflow=on  OutDataTypeStr=Inherit: Same as input
  b(76) : Gain  Gain=-2.8914777875554402e-07  ParamDataTypeStr=double  RndMeth=Nearest  SaturateOnIntegerOverflow=on  OutDataTypeStr=Inherit: Same as input
  b(77) : Gain  Gain=0.0039010037547926465  ParamDataTypeStr=double  RndMeth=Nearest  SaturateOnIntegerOverflow=on  OutDataTypeStr=Inherit: Same as input
  b(78) : Gain  Gain=-0.0040029332081024669  ParamDataTypeStr=double  RndMeth=Nearest  SaturateOnIntegerOverflow=on  OutDataTypeStr=Inherit: Same as input
  b(79) : Gain  Gain=0.0014942521610644595  ParamDataTypeStr=double  RndMeth=Nearest  SaturateOnIntegerOverflow=on  OutDataTypeStr=Inherit: Same as input
  b(8) : Gain  Gain=0.002993986641238823  ParamDataTypeStr=double  RndMeth=Nearest  SaturateOnIntegerOverflow=on  OutDataTypeStr=Inherit: Same as input
  b(80) : Gain  Gain=0.001967203062125656  ParamDataTypeStr=double  RndMeth=Nearest  SaturateOnIntegerOverflow=on  OutDataTypeStr=Inherit: Same as input
  b(9) : Gain  Gain=-0.0059345211567351126  ParamDataTypeStr=double  RndMeth=Nearest  SaturateOnIntegerOverflow=on  OutDataTypeStr=Inherit: Same as input
  Output : Outport
  wires:
  Input/1 -> b(1)/1, BodyDelay2/1
  b(1)/1 -> BodyLSum2/2
  BodyDelay2/1 -> b(2)/1, BodyDelay3/1
  b(2)/1 -> BodyLSum2/1
  BodyLSum2/1 -> BodyLSum3/2
  BodyDelay3/1 -> b(3)/1, BodyDelay4/1
  b(3)/1 -> BodyLSum3/1
  BodyLSum3/1 -> BodyLSum4/2
  BodyDelay4/1 -> b(4)/1, BodyDelay5/1
  b(4)/1 -> BodyLSum4/1
  BodyLSum4/1 -> BodyLSum5/2
  BodyDelay5/1 -> b(5)/1, BodyDelay6/1
  b(5)/1 -> BodyLSum5/1
  BodyLSum5/1 -> BodyLSum6/2
  BodyDelay6/1 -> b(6)/1, BodyDelay7/1
  b(6)/1 -> BodyLSum6/1
  BodyLSum6/1 -> BodyLSum7/2
  BodyDelay7/1 -> b(7)/1, BodyDelay8/1
  b(7)/1 -> BodyLSum7/1
  BodyLSum7/1 -> BodyLSum8/2
  BodyDelay8/1 -> b(8)/1, BodyDelay9/1
  b(8)/1 -> BodyLSum8/1
  BodyLSum8/1 -> BodyLSum9/2
  BodyDelay9/1 -> b(9)/1, BodyDelay10/1
  b(9)/1 -> BodyLSum9/1
  BodyLSum9/1 -> BodyLSum10/2
  BodyDelay10/1 -> b(10)/1, BodyDelay11/1
  b(10)/1 -> BodyLSum10/1
  BodyLSum10/1 -> BodyLSum11/2
  BodyDelay11/1 -> b(11)/1, BodyDelay12/1
  b(11)/1 -> BodyLSum11/1
  BodyLSum11/1 -> BodyLSum12/2
  BodyDelay12/1 -> b(12)/1, BodyDelay13/1
  b(12)/1 -> BodyLSum12/1
  BodyLSum12/1 -> BodyLSum13/2
  BodyDelay13/1 -> b(13)/1, BodyDelay14/1
  b(13)/1 -> BodyLSum13/1
  BodyLSum13/1 -> BodyLSum14/2
  BodyDelay14/1 -> b(14)/1, BodyDelay15/1
  b(14)/1 -> BodyLSum14/1
  BodyLSum14/1 -> BodyLSum15/2
  BodyDelay15/1 -> b(15)/1, BodyDelay16/1
  b(15)/1 -> BodyLSum15/1
  BodyLSum15/1 -> BodyLSum16/2
  BodyDelay16/1 -> b(16)/1, BodyDelay17/1
  b(16)/1 -> BodyLSum16/1
  BodyLSum16/1 -> BodyLSum17/2
  BodyDelay17/1 -> b(17)/1, BodyDelay18/1
  b(17)/1 -> BodyLSum17/1
  BodyLSum17/1 -> BodyLSum18/2
  BodyDelay18/1 -> b(18)/1, BodyDelay19/1
  b(18)/1 -> BodyLSum18/1
  BodyLSum18/1 -> BodyLSum19/2
  BodyDelay19/1 -> b(19)/1, BodyDelay20/1
  b(19)/1 -> BodyLSum19/1
  BodyLSum19/1 -> BodyLSum20/2
  BodyDelay20/1 -> b(20)/1, BodyDelay21/1
  b(20)/1 -> BodyLSum20/1
  BodyLSum20/1 -> BodyLSum21/2
  BodyDelay21/1 -> b(21)/1, BodyDelay22/1
  b(21)/1 -> BodyLSum21/1
  BodyLSum21/1 -> BodyLSum22/2
  BodyDelay22/1 -> b(22)/1, BodyDelay23/1
  b(22)/1 -> BodyLSum22/1
  BodyLSum22/1 -> BodyLSum23/2
  BodyDelay23/1 -> b(23)/1, BodyDelay24/1
  b(23)/1 -> BodyLSum23/1
  BodyLSum23/1 -> BodyLSum24/2
  BodyDelay24/1 -> b(24)/1, BodyDelay25/1
  b(24)/1 -> BodyLSum24/1
  BodyLSum24/1 -> BodyLSum25/2
  BodyDelay25/1 -> b(25)/1, BodyDelay26/1
  b(25)/1 -> BodyLSum25/1
  BodyLSum25/1 -> BodyLSum26/2
  BodyDelay26/1 -> b(26)/1, BodyDelay27/1
  b(26)/1 -> BodyLSum26/1
  BodyLSum26/1 -> BodyLSum27/2
  BodyDelay27/1 -> b(27)/1, BodyDelay28/1
  b(27)/1 -> BodyLSum27/1
  BodyLSum27/1 -> BodyLSum28/2
  BodyDelay28/1 -> b(28)/1, BodyDelay29/1
  b(28)/1 -> BodyLSum28/1
  BodyLSum28/1 -> BodyLSum29/2
  BodyDelay29/1 -> b(29)/1, BodyDelay30/1
  b(29)/1 -> BodyLSum29/1
  BodyLSum29/1 -> BodyLSum30/2
  BodyDelay30/1 -> b(30)/1, BodyDelay31/1
  b(30)/1 -> BodyLSum30/1
  BodyLSum30/1 -> BodyLSum31/2
  BodyDelay31/1 -> b(31)/1, BodyDelay32/1
  b(31)/1 -> BodyLSum31/1
  BodyLSum31/1 -> BodyLSum32/2
  BodyDelay32/1 -> b(32)/1, BodyDelay33/1
  b(32)/1 -> BodyLSum32/1
  BodyLSum32/1 -> BodyLSum33/2
  BodyDelay33/1 -> b(33)/1, BodyDelay34/1
  b(33)/1 -> BodyLSum33/1
  BodyLSum33/1 -> BodyLSum34/2
  BodyDelay34/1 -> b(34)/1, BodyDelay35/1
  b(34)/1 -> BodyLSum34/1
  BodyLSum34/1 -> BodyLSum35/2
  BodyDelay35/1 -> b(35)/1, BodyDelay36/1
  b(35)/1 -> BodyLSum35/1
  BodyLSum35/1 -> BodyLSum36/2
  BodyDelay36/1 -> b(36)/1, BodyDelay37/1
  b(36)/1 -> BodyLSum36/1
  BodyLSum36/1 -> BodyLSum37/2
  BodyDelay37/1 -> b(37)/1, BodyDelay38/1
  b(37)/1 -> BodyLSum37/1
  BodyLSum37/1 -> BodyLSum38/2
  BodyDelay38/1 -> b(38)/1, BodyDelay39/1
  b(38)/1 -> BodyLSum38/1
  BodyLSum38/1 -> BodyLSum39/2
  BodyDelay39/1 -> b(39)/1, BodyDelay40/1
  b(39)/1 -> BodyLSum39/1
  BodyLSum39/1 -> BodyLSum40/2
  BodyDelay40/1 -> BodyLSum40/1, BodyDelay41/1
  BodyLSum40/1 -> BodyLSum41/2
  BodyDelay41/1 -> BodyLSum41/1, BodyDelay42/1
  BodyLSum41/1 -> BodyLSum42/2
  BodyDelay42/1 -> b(42)/1, BodyDelay43/1
  b(42)/1 -> BodyLSum42/1
  BodyLSum42/1 -> BodyLSum43/2
  BodyDelay43/1 -> b(43)/1, BodyDelay44/1
  b(43)/1 -> BodyLSum43/1
  BodyLSum43/1 -> BodyLSum44/2
  BodyDelay44/1 -> b(44)/1, BodyDelay45/1
  b(44)/1 -> BodyLSum44/1
  BodyLSum44/1 -> BodyLSum45/2
  BodyDelay45/1 -> b(45)/1, BodyDelay46/1
  b(45)/1 -> BodyLSum45/1
  BodyLSum45/1 -> BodyLSum46/2
  BodyDelay46/1 -> b(46)/1, BodyDelay47/1
  b(46)/1 -> BodyLSum46/1
  BodyLSum46/1 -> BodyLSum47/2
  BodyDelay47/1 -> b(47)/1, BodyDelay48/1
  b(47)/1 -> BodyLSum47/1
  BodyLSum47/1 -> BodyLSum48/2
  BodyDelay48/1 -> b(48)/1, BodyDelay49/1
  b(48)/1 -> BodyLSum48/1
  BodyLSum48/1 -> BodyLSum49/2
  BodyDelay49/1 -> b(49)/1, BodyDelay50/1
  b(49)/1 -> BodyLSum49/1
  BodyLSum49/1 -> BodyLSum50/2
  BodyDelay50/1 -> b(50)/1, BodyDelay51/1
  b(50)/1 -> BodyLSum50/1
  BodyLSum50/1 -> BodyLSum51/2
  BodyDelay51/1 -> b(51)/1, BodyDelay52/1
  b(51)/1 -> BodyLSum51/1
  BodyLSum51/1 -> BodyLSum52/2
  BodyDelay52/1 -> b(52)/1, BodyDelay53/1
  b(52)/1 -> BodyLSum52/1
  BodyLSum52/1 -> BodyLSum53/2
  BodyDelay53/1 -> b(53)/1, BodyDelay54/1
  b(53)/1 -> BodyLSum53/1
  BodyLSum53/1 -> BodyLSum54/2
  BodyDelay54/1 -> b(54)/1, BodyDelay55/1
  b(54)/1 -> BodyLSum54/1
  BodyLSum54/1 -> BodyLSum55/2
  BodyDelay55/1 -> b(55)/1, BodyDelay56/1
  b(55)/1 -> BodyLSum55/1
  BodyLSum55/1 -> BodyLSum56/2
  BodyDelay56/1 -> b(56)/1, BodyDelay57/1
  b(56)/1 -> BodyLSum56/1
  BodyLSum56/1 -> BodyLSum57/2
  BodyDelay57/1 -> b(57)/1, BodyDelay58/1
  b(57)/1 -> BodyLSum57/1
  BodyLSum57/1 -> BodyLSum58/2
  BodyDelay58/1 -> b(58)/1, BodyDelay59/1
  b(58)/1 -> BodyLSum58/1
  BodyLSum58/1 -> BodyLSum59/2
  BodyDelay59/1 -> b(59)/1, BodyDelay60/1
  b(59)/1 -> BodyLSum59/1
  BodyLSum59/1 -> BodyLSum60/2
  BodyDelay60/1 -> b(60)/1, BodyDelay61/1
  b(60)/1 -> BodyLSum60/1
  BodyLSum60/1 -> BodyLSum61/2
  BodyDelay61/1 -> b(61)/1, BodyDelay62/1
  b(61)/1 -> BodyLSum61/1
  BodyLSum61/1 -> BodyLSum62/2
  BodyDelay62/1 -> b(62)/1, BodyDelay63/1
  b(62)/1 -> BodyLSum62/1
  BodyLSum62/1 -> BodyLSum63/2
  BodyDelay63/1 -> b(63)/1, BodyDelay64/1
  b(63)/1 -> BodyLSum63/1
  BodyLSum63/1 -> BodyLSum64/2
  BodyDelay64/1 -> b(64)/1, BodyDelay65/1
  b(64)/1 -> BodyLSum64/1
  BodyLSum64/1 -> BodyLSum65/2
  BodyDelay65/1 -> b(65)/1, BodyDelay66/1
  b(65)/1 -> BodyLSum65/1
  BodyLSum65/1 -> BodyLSum66/2
  BodyDelay66/1 -> b(66)/1, BodyDelay67/1
  b(66)/1 -> BodyLSum66/1
  BodyLSum66/1 -> BodyLSum67/2
  BodyDelay67/1 -> b(67)/1, BodyDelay68/1
  b(67)/1 -> BodyLSum67/1
  BodyLSum67/1 -> BodyLSum68/2
  BodyDelay68/1 -> b(68)/1, BodyDelay69/1
  b(68)/1 -> BodyLSum68/1
  BodyLSum68/1 -> BodyLSum69/2
  BodyDelay69/1 -> b(69)/1, BodyDelay70/1
  b(69)/1 -> BodyLSum69/1
  BodyLSum69/1 -> BodyLSum70/2
  BodyDelay70/1 -> b(70)/1, BodyDelay71/1
  b(70)/1 -> BodyLSum70/1
  BodyLSum70/1 -> BodyLSum71/2
  BodyDelay71/1 -> b(71)/1, BodyDelay72/1
  b(71)/1 -> BodyLSum71/1
  BodyLSum71/1 -> BodyLSum72/2
  BodyDelay72/1 -> b(72)/1, BodyDelay73/1
  b(72)/1 -> BodyLSum72/1
  BodyLSum72/1 -> BodyLSum73/2
  BodyDelay73/1 -> b(73)/1, BodyDelay74/1
  b(73)/1 -> BodyLSum73/1
  BodyLSum73/1 -> BodyLSum74/2
  BodyDelay74/1 -> b(74)/1, BodyDelay75/1
  b(74)/1 -> BodyLSum74/1
  BodyLSum74/1 -> BodyLSum75/2
  BodyDelay75/1 -> b(75)/1, BodyDelay76/1
  b(75)/1 -> BodyLSum75/1
  BodyLSum75/1 -> BodyLSum76/2
  BodyDelay76/1 -> b(76)/1, BodyDelay77/1
  b(76)/1 -> BodyLSum76/1
  BodyLSum76/1 -> BodyLSum77/2
  BodyDelay77/1 -> b(77)/1, BodyDelay78/1
  b(77)/1 -> BodyLSum77/1
  BodyLSum77/1 -> BodyLSum78/2
  BodyDelay78/1 -> b(78)/1, BodyDelay79/1
  b(78)/1 -> BodyLSum78/1
  BodyLSum78/1 -> BodyLSum79/2
  BodyDelay79/1 -> b(79)/1, BodyDelay80/1
  b(79)/1 -> BodyLSum79/1
  BodyLSum79/1 -> BodyLSum80/1
  BodyDelay80/1 -> b(80)/1
  b(80)/1 -> BodyLSum80/2
  BodyLSum80/1 -> Output/1

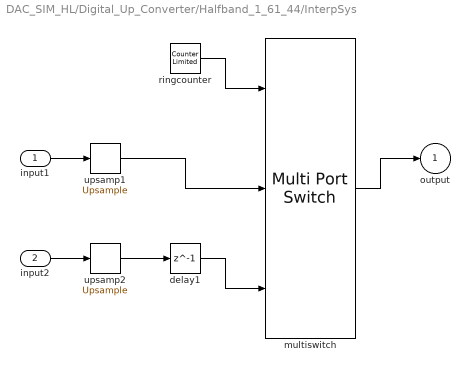
== system DAC_SIM_HL/Digital_Up_Converter/Halfband_1_61_44/InterpSys ==
  input1 : Inport
  input2 : Inport  Port=2
  delay1 : Delay  DelayLength=1
  multiswitch : MultiPortSwitch  DataPortOrder=Zero-based contiguous  Inputs=2  zeroidx=on  SaturateOnIntegerOverflow=on
  ringcounter : simulink/Sources/Counter Limited  uplimit=1  tsamp=-1
  upsamp1 : dspsigops/Upsample  N=2  phase=0  RateOptions=Allow multirate processing  ic=0  mode=Unused parameter value
  upsamp2 : dspsigops/Upsample  N=2  phase=0  RateOptions=Allow multirate processing  ic=0  mode=Unused parameter value
  output : Outport
  wires:
  ringcounter/1 -> multiswitch/1
  input1/1 -> upsamp1/1
  upsamp1/1 -> multiswitch/2
  input2/1 -> upsamp2/1
  upsamp2/1 -> delay1/1
  delay1/1 -> multiswitch/3
  multiswitch/1 -> output/1
